simulink subsystem "Burnout_Delay_Deployment"  (R2023b)
settings: Solver=VariableStepAuto  StartTime=0.0  StopTime=10.0  RelTol=1e-3
settings Model: Creator=thatf  LastModifiedBy=thatf

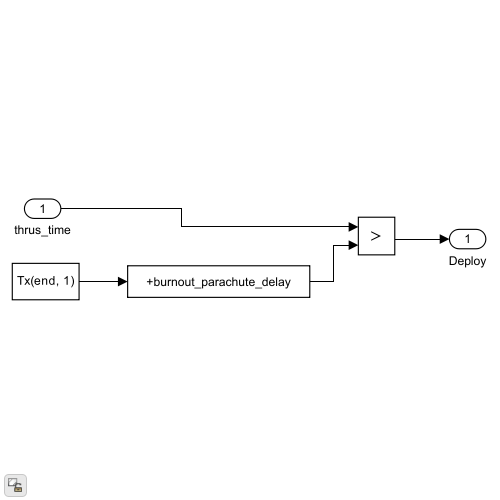
[thumbnail: Simulink's stored preview of the top-level diagram]
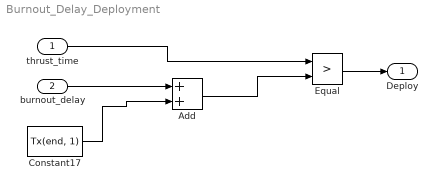
== system Burnout_Delay_Deployment ==
  thrust_time : Inport
  burnout_delay : Inport  Port=2
  Add : Sum
  Constant17 : Constant  Value=Tx(end, 1)
  Equal : RelationalOperator  Operator=>  OutDataTypeStr=boolean  RndMeth=Simplest  InputSameDT=off
  Deploy : Outport
  wires:
  Add/1 -> Equal/2
  Constant17/1 -> Add/2
  thrust_time/1 -> Equal/1
  Equal/1 -> Deploy/1
  burnout_delay/1 -> Add/1
